simulink model "cssim_tt_demo"  (Simulink 5.1)
settings: Solver=ode45  StartTime=0.0  StopTime=0.5  RelTol=1e-3
libraries: truetime x1
settings Model: LastModifiedBy=Administrator  SaveFormat=StructureWithTime  LimitDataPoints=off  MaxDataPoints=100000  BooleanDataType=on  ProdHWDeviceType=Microprocessor  RTWOptions="-aEnforceIntegerDowncast=1 -aExtMode=0 -aExtModeTesting=0 -aFoldNonRolledExpr=1 -aForceParamTrailComments=0 -aGenerateComments=1 -aGenerateReport=0 -aIgnoreCustomStorageClasses=0 -aIncDataTypeInIds=0 -aIncHierarchyInIds=0 -aInlineInvariantSignals=0 -aInlinedPrmAccess=\"Literals\" -aLocalBlockOutputs=1 -aLogVarNameModifier=\"rt_\" -aMaxRTWIdLen=31 -aPrefixModelToSubsysFcnNames=1 -aRTWVerbose=1 -aRollThreshold=5 -aShowEliminatedStatements=0"

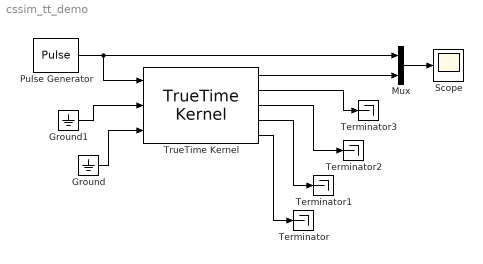
== system cssim_tt_demo ==
  Ground : Ground
  Ground1 : Ground
  Mux : Mux  Inputs=2
  Pulse Generator : DiscretePulseGenerator  PulseType=Time based  Amplitude=10  Period=1/10  PulseWidth=50
  Scope : Scope
      settings: YMin=-10  YMax=20
  Terminator{,1..3} (4 alike) : Terminator
  TrueTime Kernel : truetime/TrueTime Kernel  sfun=simple_init  args=0  battery=off  clockdrift=0  clockoffset=0
  wires:
  TrueTime Kernel/3 -> Terminator2/1
  TrueTime Kernel/5 -> Terminator/1
  TrueTime Kernel/4 -> Terminator1/1
  Ground/1 -> TrueTime Kernel/3
  Ground1/1 -> TrueTime Kernel/2
  Pulse Generator/1 -> TrueTime Kernel/1, Mux/1
  Mux/1 -> Scope/1
  TrueTime Kernel/1 -> Mux/2
  TrueTime Kernel/2 -> Terminator3/1
